simulink library "vfod_testing"  (R2021b)
settings: Solver=VariableStepAuto  StartTime=0.0  StopTime=10.0  RelTol=1e-3
libraries: fod_v2 x76
settings Model: Creator=Aleksei  LastModifiedBy=Aleksei

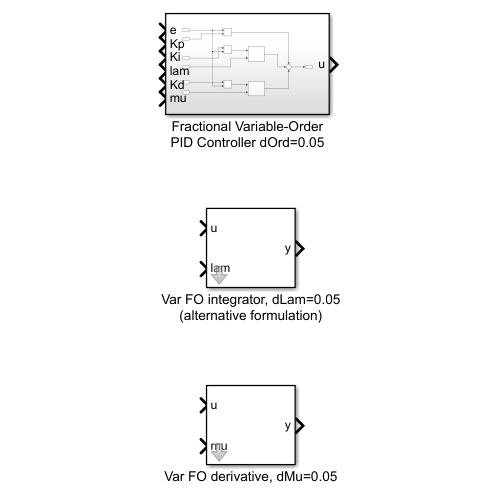
[thumbnail: Simulink's stored preview of the top-level diagram]
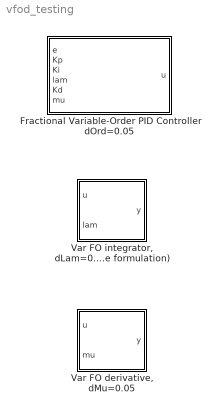
== system vfod_testing ==
  Fractional Variable-Order PID Controller dOrd=0.05 : Subsystem
  "Var FO derivative, dMu=0.05" : Subsystem  mask{freqrange=[0.001; 1000], approxorder=5}
      mask prompts: freqrange "Approximation frequency range [rad/s]"; approxorder "Oustaloup recursive filter order N"
  "Var FO integrator, dLam=0.05 (alternative formulation)" : Subsystem  mask{freqrange=[0.001; 1000], approxorder=5}
      mask prompts: freqrange "Approximation frequency range [rad/s]"; approxorder "Oustaloup recursive filter order N"

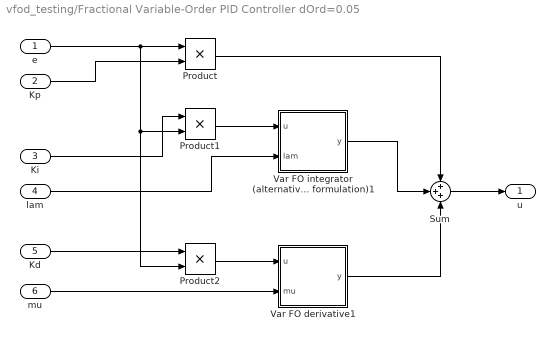
== system vfod_testing/Fractional Variable-Order PID Controller dOrd=0.05 ==
  e : Inport
  Kp : Inport  Port=2
  Ki : Inport  Port=3
  lam : Inport  Port=4
  Kd : Inport  Port=5
  mu : Inport  Port=6
  Product : Product
  Product1 : Product
  Product2 : Product
  Sum : Sum  Inputs=+++
  Var FO derivative1 : Subsystem  mask{freqrange=[0.001; 1000], approxorder=5}
      mask prompts: freqrange "Approximation frequency range [rad/s]"; approxorder "Oustaloup recursive filter order N"
  Var FO integrator (alternative formulation)1 : Subsystem  mask{freqrange=[0.001; 1000], approxorder=5}
      mask prompts: freqrange "Approximation frequency range [rad/s]"; approxorder "Oustaloup recursive filter order N"
  u : Outport
  wires:
  Var FO integrator (alternative formulation)1/1(y) -> Sum/2
  Kp/1 -> Product/2
  e/1 -> Product2/2, Product1/2, Product/1
  Product/1 -> Sum/1
  Var FO derivative1/1(y) -> Sum/3
  Sum/1 -> u/1
  Product1/1 -> Var FO integrator (alternative formulation)1/1(u)
  Ki/1 -> Product1/1
  lam/1 -> Var FO integrator (alternative formulation)1/2(lam)
  Kd/1 -> Product2/1
  mu/1 -> Var FO derivative1/2(mu)
  Product2/1 -> Var FO derivative1/1(u)

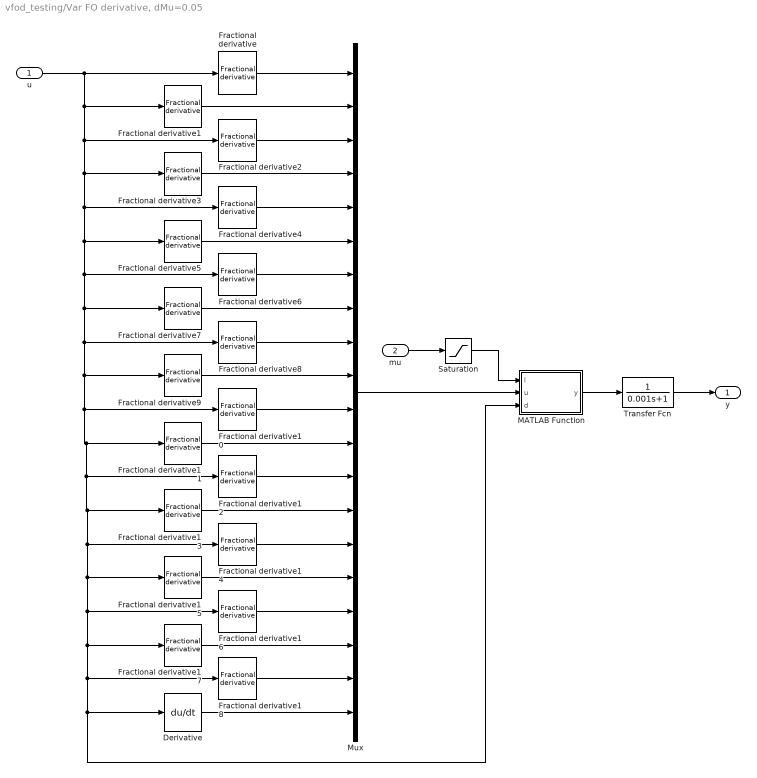
== system vfod_testing/Var FO derivative, dMu=0.05 ==
  u : Inport
  mu : Inport  Port=2
  Derivative : Derivative
  Fractional derivative : fod_v2/Fractional derivative  gam=0.05  ww=freqrange  n=approxorder  nFod=off
  Fractional derivative1 : fod_v2/Fractional derivative  gam=0.1  ww=freqrange  n=approxorder  nFod=off
  Fractional derivative10 : fod_v2/Fractional derivative  gam=0.55  ww=freqrange  n=approxorder  nFod=off
  Fractional derivative11 : fod_v2/Fractional derivative  gam=0.6  ww=freqrange  n=approxorder  nFod=off
  Fractional derivative12 : fod_v2/Fractional derivative  gam=0.65  ww=freqrange  n=approxorder  nFod=off
  Fractional derivative13 : fod_v2/Fractional derivative  gam=0.7  ww=freqrange  n=approxorder  nFod=off
  Fractional derivative14 : fod_v2/Fractional derivative  gam=0.75  ww=freqrange  n=approxorder  nFod=off
  Fractional derivative15 : fod_v2/Fractional derivative  gam=0.8  ww=freqrange  n=approxorder  nFod=off
  Fractional derivative16 : fod_v2/Fractional derivative  gam=0.85  ww=freqrange  n=approxorder  nFod=off
  Fractional derivative17 : fod_v2/Fractional derivative  gam=0.9  ww=freqrange  n=approxorder  nFod=off
  Fractional derivative18 : fod_v2/Fractional derivative  gam=0.95  ww=freqrange  n=approxorder  nFod=off
  Fractional derivative2 : fod_v2/Fractional derivative  gam=0.15  ww=freqrange  n=approxorder  nFod=off
  Fractional derivative3 : fod_v2/Fractional derivative  gam=0.2  ww=freqrange  n=approxorder  nFod=off
  Fractional derivative4 : fod_v2/Fractional derivative  gam=0.25  ww=freqrange  n=approxorder  nFod=off
  Fractional derivative5 : fod_v2/Fractional derivative  gam=0.3  ww=freqrange  n=approxorder  nFod=off
  Fractional derivative6 : fod_v2/Fractional derivative  gam=0.35  ww=freqrange  n=approxorder  nFod=off
  Fractional derivative7 : fod_v2/Fractional derivative  gam=0.4  ww=freqrange  n=approxorder  nFod=off
  Fractional derivative8 : fod_v2/Fractional derivative  gam=0.45  ww=freqrange  n=approxorder  nFod=off
  Fractional derivative9 : fod_v2/Fractional derivative  gam=0.5  ww=freqrange  n=approxorder  nFod=off
  MATLAB Function : MATLAB Function  TreatAsAtomicUnit=on
  Mux : Mux  Inputs=20
  Saturation : Saturate  UpperLimit=1  LowerLimit=0
  Transfer Fcn : TransferFcn  Denominator=[0.001 1]
  y : Outport
  wires:
  Fractional derivative/1 -> Mux/1
  Fractional derivative11/1 -> Mux/12
  Fractional derivative6/1 -> Mux/7
  Fractional derivative5/1 -> Mux/6
  Fractional derivative8/1 -> Mux/9
  Fractional derivative1/1 -> Mux/2
  Fractional derivative12/1 -> Mux/13
  Fractional derivative10/1 -> Mux/11
  Fractional derivative14/1 -> Mux/15
  Fractional derivative7/1 -> Mux/8
  Fractional derivative17/1 -> Mux/18
  Fractional derivative2/1 -> Mux/3
  Fractional derivative3/1 -> Mux/4
  Derivative/1 -> Mux/20
  Fractional derivative16/1 -> Mux/17
  Fractional derivative4/1 -> Mux/5
  Mux/1 -> MATLAB Function/2(u)
  Fractional derivative15/1 -> Mux/16
  MATLAB Function/1(y) -> Transfer Fcn/1
  Fractional derivative9/1 -> Mux/10
  Fractional derivative18/1 -> Mux/19
  Fractional derivative13/1 -> Mux/14
  mu/1 -> Saturation/1
  u/1 -> Fractional derivative7/1, MATLAB Function/3(d), Derivative/1, Fractional derivative18/1, Fractional derivative17/1, Fractional derivative16/1, Fractional derivative15/1, Fractional derivative14/1, Fractional derivative13/1, Fractional derivative12/1, Fractional derivative11/1, Fractional derivative10/1, Fractional derivative9/1, Fractional derivative8/1, Fractional derivative6/1, Fractional derivative5/1, Fractional derivative4/1, Fractional derivative3/1, Fractional derivative2/1, Fractional derivative1/1, Fractional derivative/1
  Saturation/1 -> MATLAB Function/1(l)
  Transfer Fcn/1 -> y/1

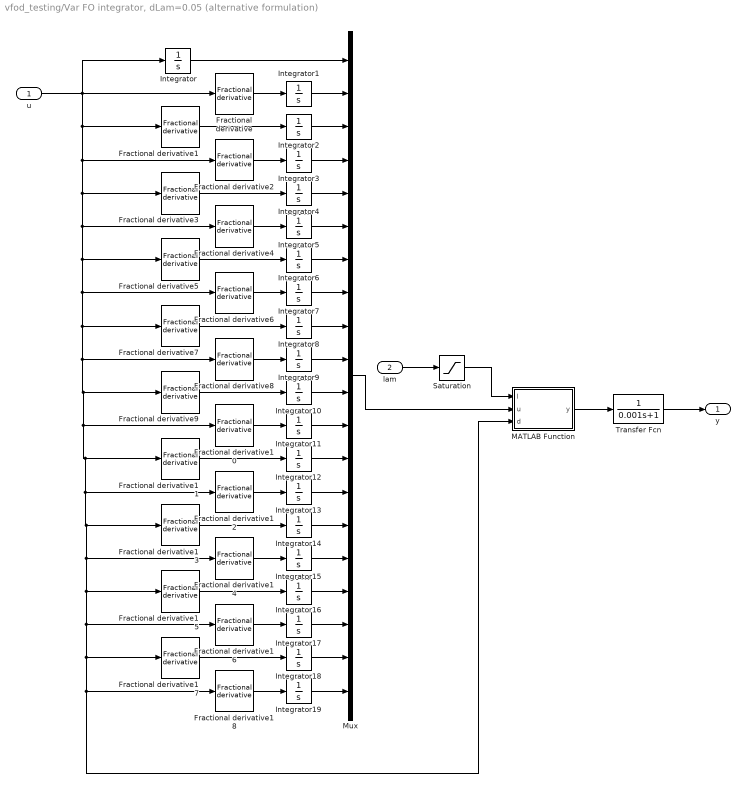
== system vfod_testing/Var FO integrator, dLam=0.05 (alternative formulation) ==
  u : Inport
  lam : Inport  Port=2
  Fractional derivative : fod_v2/Fractional derivative  gam=0.05  ww=freqrange  n=approxorder  nFod=off
  Fractional derivative1 : fod_v2/Fractional derivative  gam=0.1  ww=freqrange  n=approxorder  nFod=off
  Fractional derivative10 : fod_v2/Fractional derivative  gam=0.55  ww=freqrange  n=approxorder  nFod=off
  Fractional derivative11 : fod_v2/Fractional derivative  gam=0.6  ww=freqrange  n=approxorder  nFod=off
  Fractional derivative12 : fod_v2/Fractional derivative  gam=0.65  ww=freqrange  n=approxorder  nFod=off
  Fractional derivative13 : fod_v2/Fractional derivative  gam=0.7  ww=freqrange  n=approxorder  nFod=off
  Fractional derivative14 : fod_v2/Fractional derivative  gam=0.75  ww=freqrange  n=approxorder  nFod=off
  Fractional derivative15 : fod_v2/Fractional derivative  gam=0.8  ww=freqrange  n=approxorder  nFod=off
  Fractional derivative16 : fod_v2/Fractional derivative  gam=0.85  ww=freqrange  n=approxorder  nFod=off
  Fractional derivative17 : fod_v2/Fractional derivative  gam=0.9  ww=freqrange  n=approxorder  nFod=off
  Fractional derivative18 : fod_v2/Fractional derivative  gam=0.95  ww=freqrange  n=approxorder  nFod=off
  Fractional derivative2 : fod_v2/Fractional derivative  gam=0.15  ww=freqrange  n=approxorder  nFod=off
  Fractional derivative3 : fod_v2/Fractional derivative  gam=0.2  ww=freqrange  n=approxorder  nFod=off
  Fractional derivative4 : fod_v2/Fractional derivative  gam=0.25  ww=freqrange  n=approxorder  nFod=off
  Fractional derivative5 : fod_v2/Fractional derivative  gam=0.3  ww=freqrange  n=approxorder  nFod=off
  Fractional derivative6 : fod_v2/Fractional derivative  gam=0.35  ww=freqrange  n=approxorder  nFod=off
  Fractional derivative7 : fod_v2/Fractional derivative  gam=0.4  ww=freqrange  n=approxorder  nFod=off
  Fractional derivative8 : fod_v2/Fractional derivative  gam=0.45  ww=freqrange  n=approxorder  nFod=off
  Fractional derivative9 : fod_v2/Fractional derivative  gam=0.5  ww=freqrange  n=approxorder  nFod=off
  Integrator{,1..19} (20 alike) : Integrator
  MATLAB Function : MATLAB Function  TreatAsAtomicUnit=on
  Mux : Mux  Inputs=20
  Saturation : Saturate  UpperLimit=1  LowerLimit=0
  Transfer Fcn : TransferFcn  Denominator=[0.001 1]
  y : Outport
  wires:
  Mux/1 -> MATLAB Function/2(u)
  MATLAB Function/1(y) -> Transfer Fcn/1
  lam/1 -> Saturation/1
  u/1 -> Fractional derivative7/1, MATLAB Function/3(d), Fractional derivative18/1, Fractional derivative17/1, Fractional derivative16/1, Fractional derivative15/1, Fractional derivative14/1, Fractional derivative13/1, Fractional derivative12/1, Fractional derivative11/1, Fractional derivative10/1, Fractional derivative9/1, Fractional derivative8/1, Fractional derivative6/1, Fractional derivative5/1, Fractional derivative4/1, Fractional derivative3/1, Fractional derivative2/1, Fractional derivative1/1, Integrator/1, Fractional derivative/1
  Saturation/1 -> MATLAB Function/1(l)
  Transfer Fcn/1 -> y/1
  Integrator/1 -> Mux/1
  Fractional derivative/1 -> Integrator1/1
  Integrator1/1 -> Mux/2
  Integrator2/1 -> Mux/3
  Fractional derivative1/1 -> Integrator2/1
  Integrator3/1 -> Mux/4
  Fractional derivative2/1 -> Integrator3/1
  Integrator4/1 -> Mux/5
  Fractional derivative3/1 -> Integrator4/1
  Fractional derivative4/1 -> Integrator5/1
  Integrator5/1 -> Mux/6
  Fractional derivative5/1 -> Integrator6/1
  Integrator6/1 -> Mux/7
  Fractional derivative6/1 -> Integrator7/1
  Integrator7/1 -> Mux/8
  Integrator8/1 -> Mux/9
  Fractional derivative7/1 -> Integrator8/1
  Fractional derivative8/1 -> Integrator9/1
  Integrator9/1 -> Mux/10
  Integrator10/1 -> Mux/11
  Fractional derivative9/1 -> Integrator10/1
  Integrator11/1 -> Mux/12
  Fractional derivative10/1 -> Integrator11/1
  Integrator12/1 -> Mux/13
  Fractional derivative11/1 -> Integrator12/1
  Integrator13/1 -> Mux/14
  Fractional derivative12/1 -> Integrator13/1
  Integrator14/1 -> Mux/15
  Fractional derivative13/1 -> Integrator14/1
  Integrator15/1 -> Mux/16
  Fractional derivative14/1 -> Integrator15/1
  Integrator16/1 -> Mux/17
  Fractional derivative15/1 -> Integrator16/1
  Integrator17/1 -> Mux/18
  Fractional derivative16/1 -> Integrator17/1
  Integrator18/1 -> Mux/19
  Fractional derivative17/1 -> Integrator18/1
  Integrator19/1 -> Mux/20
  Fractional derivative18/1 -> Integrator19/1

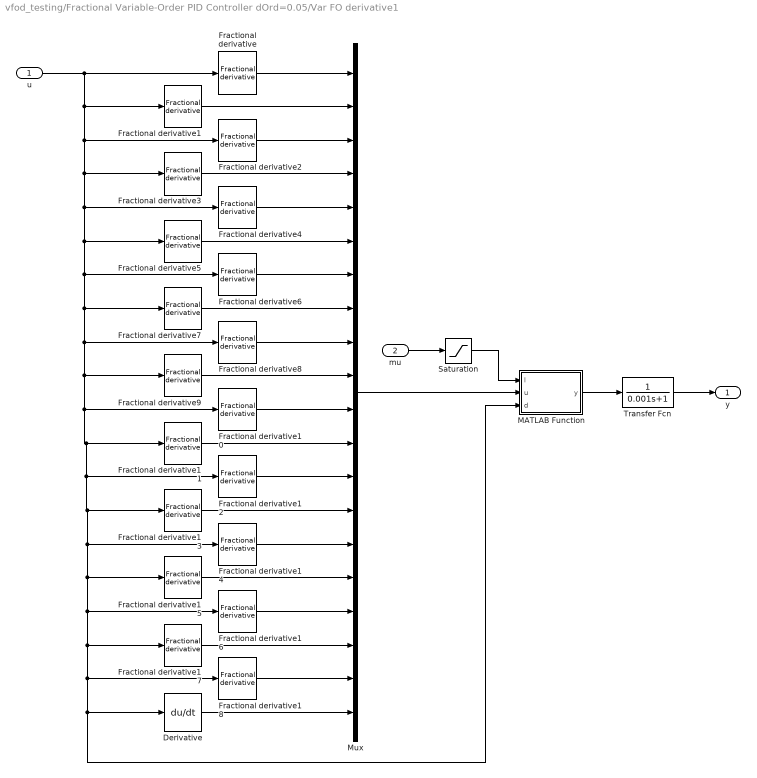
== system vfod_testing/Fractional Variable-Order PID Controller dOrd=0.05/Var FO derivative1 ==
  u : Inport
  mu : Inport  Port=2
  Derivative : Derivative
  Fractional derivative : fod_v2/Fractional derivative  gam=0.05  ww=freqrange  n=approxorder  nFod=off
  Fractional derivative1 : fod_v2/Fractional derivative  gam=0.1  ww=freqrange  n=approxorder  nFod=off
  Fractional derivative10 : fod_v2/Fractional derivative  gam=0.55  ww=freqrange  n=approxorder  nFod=off
  Fractional derivative11 : fod_v2/Fractional derivative  gam=0.6  ww=freqrange  n=approxorder  nFod=off
  Fractional derivative12 : fod_v2/Fractional derivative  gam=0.65  ww=freqrange  n=approxorder  nFod=off
  Fractional derivative13 : fod_v2/Fractional derivative  gam=0.7  ww=freqrange  n=approxorder  nFod=off
  Fractional derivative14 : fod_v2/Fractional derivative  gam=0.75  ww=freqrange  n=approxorder  nFod=off
  Fractional derivative15 : fod_v2/Fractional derivative  gam=0.8  ww=freqrange  n=approxorder  nFod=off
  Fractional derivative16 : fod_v2/Fractional derivative  gam=0.85  ww=freqrange  n=approxorder  nFod=off
  Fractional derivative17 : fod_v2/Fractional derivative  gam=0.9  ww=freqrange  n=approxorder  nFod=off
  Fractional derivative18 : fod_v2/Fractional derivative  gam=0.95  ww=freqrange  n=approxorder  nFod=off
  Fractional derivative2 : fod_v2/Fractional derivative  gam=0.15  ww=freqrange  n=approxorder  nFod=off
  Fractional derivative3 : fod_v2/Fractional derivative  gam=0.2  ww=freqrange  n=approxorder  nFod=off
  Fractional derivative4 : fod_v2/Fractional derivative  gam=0.25  ww=freqrange  n=approxorder  nFod=off
  Fractional derivative5 : fod_v2/Fractional derivative  gam=0.3  ww=freqrange  n=approxorder  nFod=off
  Fractional derivative6 : fod_v2/Fractional derivative  gam=0.35  ww=freqrange  n=approxorder  nFod=off
  Fractional derivative7 : fod_v2/Fractional derivative  gam=0.4  ww=freqrange  n=approxorder  nFod=off
  Fractional derivative8 : fod_v2/Fractional derivative  gam=0.45  ww=freqrange  n=approxorder  nFod=off
  Fractional derivative9 : fod_v2/Fractional derivative  gam=0.5  ww=freqrange  n=approxorder  nFod=off
  MATLAB Function : MATLAB Function  TreatAsAtomicUnit=on
  Mux : Mux  Inputs=20
  Saturation : Saturate  UpperLimit=1  LowerLimit=0
  Transfer Fcn : TransferFcn  Denominator=[0.001 1]
  y : Outport
  wires:
  Fractional derivative/1 -> Mux/1
  Fractional derivative11/1 -> Mux/12
  Fractional derivative6/1 -> Mux/7
  Fractional derivative5/1 -> Mux/6
  Fractional derivative8/1 -> Mux/9
  Fractional derivative1/1 -> Mux/2
  Fractional derivative12/1 -> Mux/13
  Fractional derivative10/1 -> Mux/11
  Fractional derivative14/1 -> Mux/15
  Fractional derivative7/1 -> Mux/8
  Fractional derivative17/1 -> Mux/18
  Fractional derivative2/1 -> Mux/3
  Fractional derivative3/1 -> Mux/4
  Derivative/1 -> Mux/20
  Fractional derivative16/1 -> Mux/17
  Fractional derivative4/1 -> Mux/5
  Mux/1 -> MATLAB Function/2(u)
  Fractional derivative15/1 -> Mux/16
  MATLAB Function/1(y) -> Transfer Fcn/1
  Fractional derivative9/1 -> Mux/10
  Fractional derivative18/1 -> Mux/19
  Fractional derivative13/1 -> Mux/14
  mu/1 -> Saturation/1
  u/1 -> Fractional derivative7/1, MATLAB Function/3(d), Derivative/1, Fractional derivative18/1, Fractional derivative17/1, Fractional derivative16/1, Fractional derivative15/1, Fractional derivative14/1, Fractional derivative13/1, Fractional derivative12/1, Fractional derivative11/1, Fractional derivative10/1, Fractional derivative9/1, Fractional derivative8/1, Fractional derivative6/1, Fractional derivative5/1, Fractional derivative4/1, Fractional derivative3/1, Fractional derivative2/1, Fractional derivative1/1, Fractional derivative/1
  Saturation/1 -> MATLAB Function/1(l)
  Transfer Fcn/1 -> y/1

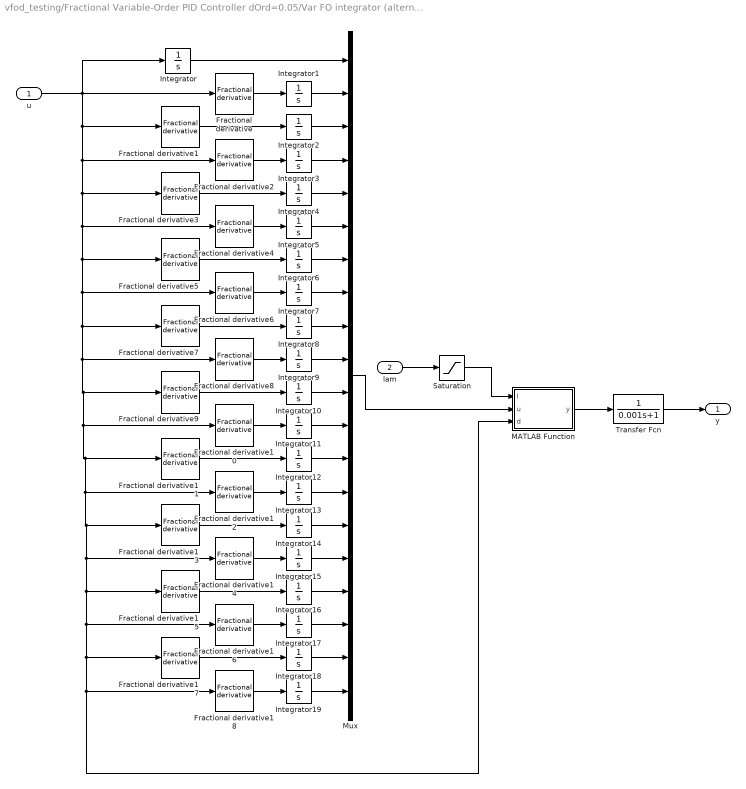
== system vfod_testing/Fractional Variable-Order PID Controller dOrd=0.05/Var FO integrator (alternative formulation)1 ==
  u : Inport
  lam : Inport  Port=2
  Fractional derivative : fod_v2/Fractional derivative  gam=0.05  ww=freqrange  n=approxorder  nFod=off
  Fractional derivative1 : fod_v2/Fractional derivative  gam=0.1  ww=freqrange  n=approxorder  nFod=off
  Fractional derivative10 : fod_v2/Fractional derivative  gam=0.55  ww=freqrange  n=approxorder  nFod=off
  Fractional derivative11 : fod_v2/Fractional derivative  gam=0.6  ww=freqrange  n=approxorder  nFod=off
  Fractional derivative12 : fod_v2/Fractional derivative  gam=0.65  ww=freqrange  n=approxorder  nFod=off
  Fractional derivative13 : fod_v2/Fractional derivative  gam=0.7  ww=freqrange  n=approxorder  nFod=off
  Fractional derivative14 : fod_v2/Fractional derivative  gam=0.75  ww=freqrange  n=approxorder  nFod=off
  Fractional derivative15 : fod_v2/Fractional derivative  gam=0.8  ww=freqrange  n=approxorder  nFod=off
  Fractional derivative16 : fod_v2/Fractional derivative  gam=0.85  ww=freqrange  n=approxorder  nFod=off
  Fractional derivative17 : fod_v2/Fractional derivative  gam=0.9  ww=freqrange  n=approxorder  nFod=off
  Fractional derivative18 : fod_v2/Fractional derivative  gam=0.95  ww=freqrange  n=approxorder  nFod=off
  Fractional derivative2 : fod_v2/Fractional derivative  gam=0.15  ww=freqrange  n=approxorder  nFod=off
  Fractional derivative3 : fod_v2/Fractional derivative  gam=0.2  ww=freqrange  n=approxorder  nFod=off
  Fractional derivative4 : fod_v2/Fractional derivative  gam=0.25  ww=freqrange  n=approxorder  nFod=off
  Fractional derivative5 : fod_v2/Fractional derivative  gam=0.3  ww=freqrange  n=approxorder  nFod=off
  Fractional derivative6 : fod_v2/Fractional derivative  gam=0.35  ww=freqrange  n=approxorder  nFod=off
  Fractional derivative7 : fod_v2/Fractional derivative  gam=0.4  ww=freqrange  n=approxorder  nFod=off
  Fractional derivative8 : fod_v2/Fractional derivative  gam=0.45  ww=freqrange  n=approxorder  nFod=off
  Fractional derivative9 : fod_v2/Fractional derivative  gam=0.5  ww=freqrange  n=approxorder  nFod=off
  Integrator{,1..19} (20 alike) : Integrator
  MATLAB Function : MATLAB Function  TreatAsAtomicUnit=on
  Mux : Mux  Inputs=20
  Saturation : Saturate  UpperLimit=1  LowerLimit=0
  Transfer Fcn : TransferFcn  Denominator=[0.001 1]
  y : Outport
  wires:
  Mux/1 -> MATLAB Function/2(u)
  MATLAB Function/1(y) -> Transfer Fcn/1
  lam/1 -> Saturation/1
  u/1 -> Fractional derivative7/1, MATLAB Function/3(d), Fractional derivative18/1, Fractional derivative17/1, Fractional derivative16/1, Fractional derivative15/1, Fractional derivative14/1, Fractional derivative13/1, Fractional derivative12/1, Fractional derivative11/1, Fractional derivative10/1, Fractional derivative9/1, Fractional derivative8/1, Fractional derivative6/1, Fractional derivative5/1, Fractional derivative4/1, Fractional derivative3/1, Fractional derivative2/1, Fractional derivative1/1, Integrator/1, Fractional derivative/1
  Saturation/1 -> MATLAB Function/1(l)
  Transfer Fcn/1 -> y/1
  Integrator/1 -> Mux/1
  Fractional derivative/1 -> Integrator1/1
  Integrator1/1 -> Mux/2
  Integrator2/1 -> Mux/3
  Fractional derivative1/1 -> Integrator2/1
  Integrator3/1 -> Mux/4
  Fractional derivative2/1 -> Integrator3/1
  Integrator4/1 -> Mux/5
  Fractional derivative3/1 -> Integrator4/1
  Fractional derivative4/1 -> Integrator5/1
  Integrator5/1 -> Mux/6
  Fractional derivative5/1 -> Integrator6/1
  Integrator6/1 -> Mux/7
  Fractional derivative6/1 -> Integrator7/1
  Integrator7/1 -> Mux/8
  Integrator8/1 -> Mux/9
  Fractional derivative7/1 -> Integrator8/1
  Fractional derivative8/1 -> Integrator9/1
  Integrator9/1 -> Mux/10
  Integrator10/1 -> Mux/11
  Fractional derivative9/1 -> Integrator10/1
  Integrator11/1 -> Mux/12
  Fractional derivative10/1 -> Integrator11/1
  Integrator12/1 -> Mux/13
  Fractional derivative11/1 -> Integrator12/1
  Integrator13/1 -> Mux/14
  Fractional derivative12/1 -> Integrator13/1
  Integrator14/1 -> Mux/15
  Fractional derivative13/1 -> Integrator14/1
  Integrator15/1 -> Mux/16
  Fractional derivative14/1 -> Integrator15/1
  Integrator16/1 -> Mux/17
  Fractional derivative15/1 -> Integrator16/1
  Integrator17/1 -> Mux/18
  Fractional derivative16/1 -> Integrator17/1
  Integrator18/1 -> Mux/19
  Fractional derivative17/1 -> Integrator18/1
  Integrator19/1 -> Mux/20
  Fractional derivative18/1 -> Integrator19/1

== matlab function vfod_testing/Var FO derivative, dMu=0.05/MATLAB Function ==
  data: l input; u input; y output size=1; d input
function y = fcn(l, u, d)

% Choice of output based on the order
% Only discrete orders supported with a step of dMu=0.05
dMu = 0.05;
myin = round(l/dMu);
if myin == 0
    y = d;
else
    y = u(myin);
end

== matlab function vfod_testing/Fractional Variable-Order PID Controller dOrd=0.05/Var FO derivative1/MATLAB Function ==
  data: l input; u input; y output size=1; d input
function y = fcn(l, u, d)

% Choice of output based on the order
% Only discrete orders supported with a step of dMu=0.05
dMu = 0.05;
myin = round(l/dMu);
if myin == 0
    y = d;
else
    y = u(myin);
end

== matlab function vfod_testing/Fractional Variable-Order PID Controller dOrd=0.05/Var FO integrator (alternative formulation)1/MATLAB Function ==
  data: l input; u input; y output size=1; d input
function y = fcn(l, u, d)

% Choice of output based on the order
% Only discrete orders supported with a step of dLam=0.05
dLam = 0.05;
myaltin = round((1-l)/dLam)+1;
% For the alternative formulation, find the correct
% input to pass based on 1-\lambda
if myaltin > 20
    y = d;
else

    y = u(myaltin);
end

== matlab function vfod_testing/Var FO integrator, dLam=0.05 (alternative formulation)/MATLAB Function ==
  data: l input; u input; y output size=1; d input
function y = fcn(l, u, d)

% Choice of output based on the order
% Only discrete orders supported with a step of dLam=0.05
dLam = 0.05;
myaltin = round((1-l)/dLam)+1;
% For the alternative formulation, find the correct
% input to pass based on 1-\lambda
if myaltin > 20
    y = d;
else

    y = u(myaltin);
end
